simulink model "satq_SATQproportions"  (R2017a)
settings: Solver=VariableStepAuto  StartTime=0.0  StopTime=50.0  RelTol=1e-3
values from neighbouring files (symbols this model uses):
  b = 0.250025    [satq_values.m]
  beta = 0.55    [satq_values.m]
  d = 0.25    [satq_values.m]
  delta = 0.3    [satq_values.m]
  epsilon = 0.8    [satq_values.m]
settings Model: Creator=rosha  LastModifiedBy=Anirudh

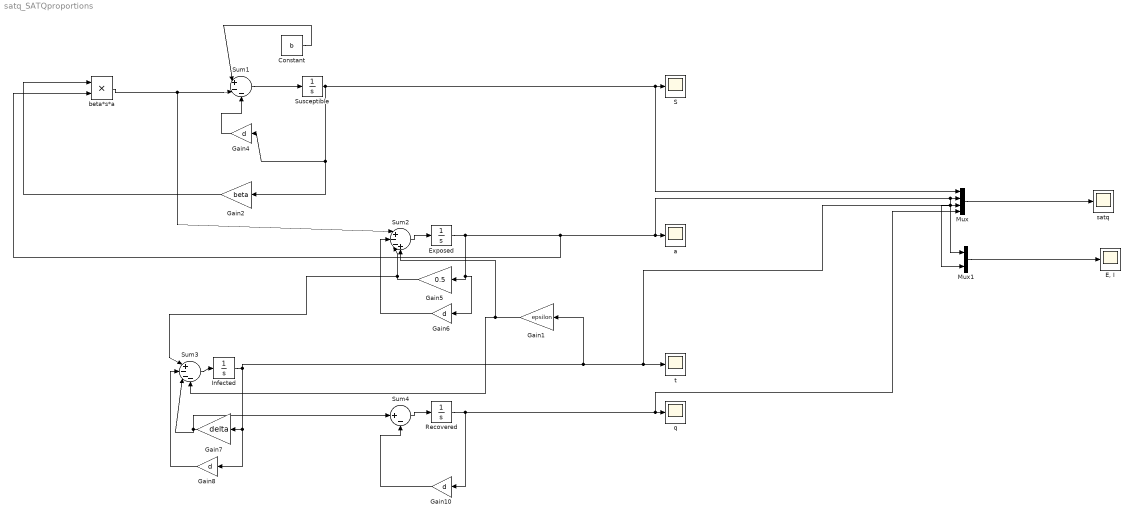
== system satq_SATQproportions ==
  Constant : Constant  Value=b
  "E, I" : Scope
  Exposed : Integrator  InitialCondition=0.250
  Gain1 : Gain  Gain=epsilon
  Gain{4,6,8,10} (4 alike) : Gain  Gain=d
  Gain2 : Gain  Gain=beta
  Gain5 : Gain  Gain=0.5
  Gain7 : Gain  Gain=delta
  Infected : Integrator  InitialCondition=0.080
  Mux : Mux
  Mux1 : Mux  Inputs=2
  Recovered : Integrator  InitialCondition=0.020
  S : Scope
  Sum1 : Sum  Inputs=|+--
  Sum2 : Sum  Inputs=|+--+
  Sum3 : Sum  Inputs=|+---
  Sum4 : Sum  Inputs=|+-
  Susceptible : Integrator  InitialCondition=0.650
  a : Scope
  beta*s*a : Product  Inputs=**
  q : Scope
  satq : Scope
  t : Scope
  wires:
  Constant/1 -> Sum1/1
  Gain7/1 -> Sum3/3, Sum4/1
  Sum4/1 -> Recovered/1
  Gain8/1 -> Sum3/2
  Infected/1 -> Gain8/1, Gain7/1, Gain1/1, Mux1/2, Mux/3, t/1
  Sum3/1 -> Infected/1
  Recovered/1 -> Gain10/1, Mux/4, q/1
  Mux1/1 -> "E, I"/1
  Exposed/1 -> Gain5/1, Gain6/1, beta*s*a/2, Mux1/1, Mux/2, a/1
  Gain5/1 -> Sum3/1, Sum2/3
  Gain10/1 -> Sum4/2
  Sum1/1 -> Susceptible/1
  Sum2/1 -> Exposed/1
  Mux/1 -> satq/1
  beta*s*a/1 -> Sum2/1, Sum1/2
  Gain4/1 -> Sum1/3
  Gain2/1 -> beta*s*a/1
  Susceptible/1 -> Gain4/1, Gain2/1, Mux/1, S/1
  Gain6/1 -> Sum2/2
  Gain1/1 -> Sum3/4, Sum2/4
